simulink model "factorial_function"  (R2021a)
settings: Solver=VariableStepAuto  StartTime=0.0  StopTime=10.0  RelTol=1e-3
settings Model: Creator=iT-User  LastModifiedBy=iT-User

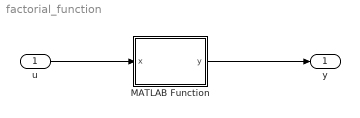
== system factorial_function ==
  u : Inport
  MATLAB Function : MATLAB Function  TreatAsAtomicUnit=on
  y : Outport
  wires:
  u/1 -> MATLAB Function/1(x)
  MATLAB Function/1(y) -> y/1

== matlab function factorial_function/MATLAB Function ==
  data: x input; y output
function y = factorial_calculator(x)
    y = 1;
    for i = 1:x
        y = y * i;
    end
end
